simulink model "pendulum_animation"  (R2018b)
settings: Solver=ode4  StartTime=0.0  StopTime=600000  FixedStep=0.01  RelTol=1e-3
undefined symbols (not defined in the file or in its folder): drawPendulum
libraries: simulink x2
settings Model: Creator=do  LastModifiedBy=do

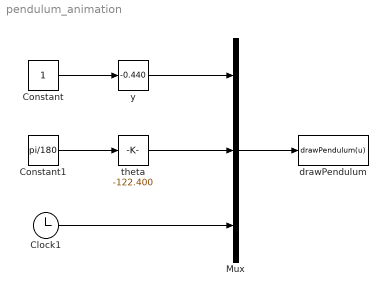
== system pendulum_animation ==
  Clock1 : Clock
  Constant : Constant
  Constant1 : Constant  Value=pi/180
  Mux : Mux  Inputs=3
  drawPendulum : MATLABFcn  MATLABFcn=drawPendulum(u)  OutputDimensions=0  Output1D=off
  theta : simulink/Math Operations/Slider Gain  gain=-122.400  low=-360  high=360
  y : simulink/Math Operations/Slider Gain  gain=-0.440  low=-1  high=1
  wires:
  Clock1/1 -> Mux/3
  theta/1 -> Mux/2
  Constant1/1 -> theta/1
  Constant/1 -> y/1
  y/1 -> Mux/1
  Mux/1 -> drawPendulum/1
